simulink model "model"  (R2021a)
settings: Solver=VariableStepAuto  StartTime=0.0  StopTime=10000  RelTol=1e-3
model workspace (MAT data in the model file):
  influence_amp = 200
  store_limit = 50
undefined symbols (not defined in the file or in its folder): DiscIntNeverNeededParam
libraries: simulink x1, pingcap x1
settings Model: Creator=tongjian  LastModifiedBy=tongjian

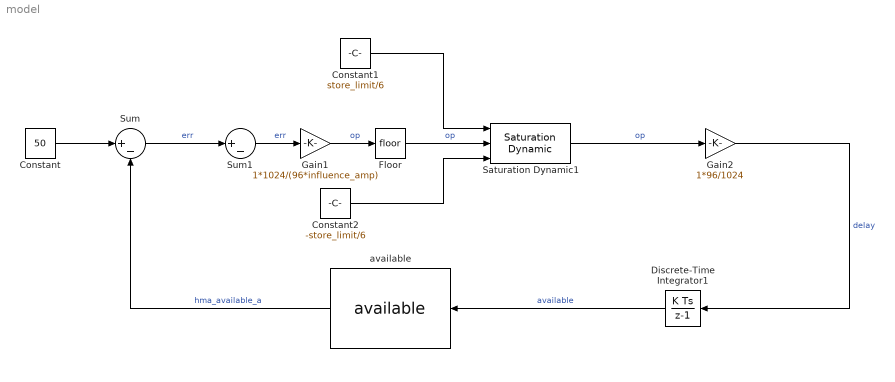
== system model ==
  Constant : Constant  Value=50
  Constant1 : Constant  Value=store_limit/6
  Constant2 : Constant  Value=-store_limit/6
  Discrete-Time Integrator1 : DiscreteIntegrator  gainval=1  InitialCondition=100  SampleTime=10  ICPrevOutput=DiscIntNeverNeededParam  ICPrevScaledInput=DiscIntNeverNeededParam
  Floor : Rounding
  Gain1 : Gain  Gain=1*1024/(96*influence_amp)  OutMin=[-3]  OutMax=[3]
  Gain2 : Gain  Gain=1*96/1024
  Saturation Dynamic1 : simulink/Discontinuities/Saturation Dynamic  OutMin=[]  OutMax=[]  OutDataTypeStr=Inherit: Same as second input  OutDataType=fixdt(1, 16)  OutScaling=2^-10  DoSatur=off
  Sum : Sum  Inputs=|+-
  Sum1 : Sum  Inputs=|+-
  available : pingcap/available  g_Ts=10  g_hma_nums_deviation_0=hma_nums_deviation_0  g_hma_dens_deviation_0=hma_dens_deviation_0  g_hma_nums_deviation_1=hma_nums_deviation_1  g_hma_dens_deviation_1=hma_dens_deviation_0  g_hma_nums_deviation_2=hma_nums_deviation_2  g_hma_dens_deviation_2=hma_dens_deviation_0  g_hma_nums_avg_0=hma_nums_avg_0  g_hma_dens_avg_0=hma_dens_avg_0  g_hma_nums_avg_1=hma_nums_avg_0  g_hma_dens_avg_1=hma_dens_avg_0  g_hma_nums_avg_2=hma_nums_avg_0  g_hma_dens_avg_2=hma_dens_avg_0  g_initial=1000
  wires:
  Constant/1 -> Sum/1
  Constant2/1 -> Saturation Dynamic1/3
  Constant1/1 -> Saturation Dynamic1/1
  Gain2/1 -> Discrete-Time Integrator1/1  "delay"
  Gain1/1 -> Floor/1  "op"
  Sum/1 -> Sum1/1  "err"
  Sum1/1 -> Gain1/1  "err"
  Discrete-Time Integrator1/1 -> available/1  "available"
  available/2 -> Sum/2  "hma_available_a"
  Floor/1 -> Saturation Dynamic1/2  "op"
  Saturation Dynamic1/1 -> Gain2/1  "op"
